simulink model "P4_Model_2"  (R2023b)
settings: Solver=VariableStepAuto  StartTime=0.0  StopTime=10.0  RelTol=1e-3
values from neighbouring files (symbols this model uses):
  C0 = 0.0041    [Finalinit.m]
  C1 = 0.000066    (= 6.6e-05)    [Finalinit.m]
  C2 = 0.5*Rho*A*Cd    (= 0.51156)    [Finalinit.m]
  Iw = 0.5*7*(r^2)    (= 0.4536)    [Finalinit.m]
  M = 1000    [Finalinit.m]
  r = 0.36    [Finalinit.m]
  rps2rpm = 60/(2*pi())    [Finalinit.m]
undefined symbols (not defined in the file or in its folder): batData, carData, motorData
libraries: slpidlib x2
settings Model: Creator=jessi  LastModifiedBy=Beye

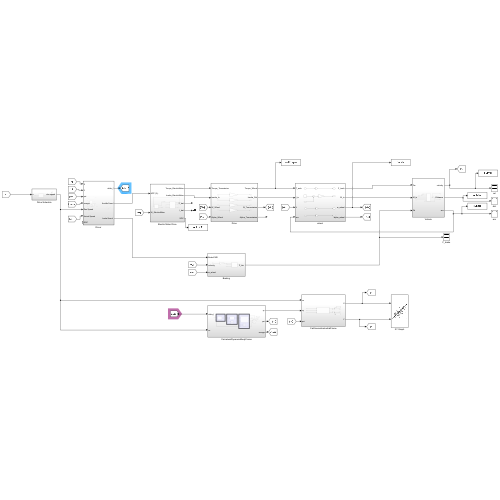
[thumbnail: Simulink's stored preview of the top-level diagram]
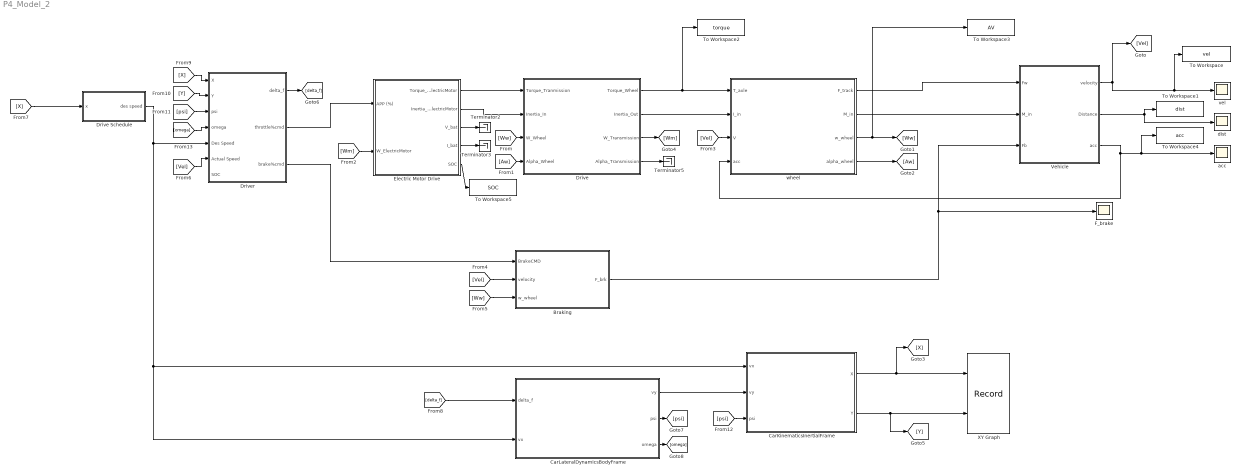
== system P4_Model_2 ==
  Braking : Subsystem
  CarKinematicsInertialFrame : Subsystem
  CarLateralDynamicsBodyFrame : Subsystem
  Drive : Subsystem
  Drive Schedule : Subsystem
  Driver : Subsystem
  Electric Motor Drive : Subsystem
  F_brake : Scope
  Terminator2 : Terminator
  Terminator3 : Terminator
  Terminator5 : Terminator
  To Workspace : ToWorkspace  VariableName=vel  SaveFormat=Timeseries  SampleTime=-1
  To Workspace1 : ToWorkspace  VariableName=dist  SaveFormat=Timeseries  SampleTime=-1
  To Workspace2 : ToWorkspace  VariableName=torque  SaveFormat=Timeseries  SampleTime=-1
  To Workspace3 : ToWorkspace  VariableName=AV  SaveFormat=Timeseries  SampleTime=-1
  To Workspace4 : ToWorkspace  VariableName=acc  SaveFormat=Timeseries  SampleTime=-1
  To Workspace5 : ToWorkspace  VariableName=SOC  SaveFormat=Timeseries  SampleTime=-1
  Vehicle : Subsystem
  XY Graph : Record  FileSettingsInternal="{\"entries\":[{\"content\":{\"excelSettings\":{\"content\":{},\"type\":\"Streamout.ExcelSettings\"}},\"type\":\"Streamout.FileSettingStorage\",\"uuid\":\"\"}],\"packageUris\":[\"http:\\/\\/schema.mathworks.com\\/mf0\\/streamout_blocks\\/R2020a\"],\"version\":\"1.0\"}"  Layout=[1 1]  SignalsInternal="{\"entries\":[{\"content\":{\"signals\":[{\"content\":{\"blockPath\":[],\"dimensions\":[1],\"domain\":\"\",\"lineColor\":\"#0072bd\",\"port\":1,\"sid\":[\"\"],\"signalID\":785,\"signalName\":\"CarKinematicsInertialFrame:1\"},\"type\":\"RecordBlkView.Signal\",\"uuid\":\"\"},{\"content\":{\"blockPath\":[],\"dimensions\":[1],\"domain\":\"\",\"lineColor\":\"#d95319\",\"port\":2,\"sid\":[\"\"],\"signalID\":789,\"signalName\":\"CarKinematicsInertialFrame:2\"},\"type\":\"RecordBlkView.Signal\",\"uuid\":\"\"}]},\"type\":\"RecordBlkView.InputSignals\",\"uuid\":\"\"}],\"packageUris\":[\"http:\\/\\/schema.mathworks.com\\/mf0\\/streamout_blocks\\/R2020a\"],\"version\":\"1.0\"}"  VisualizationBindings="{\"xyplotplugin\":{\"info\":[{\"series\":[],\"subplotID\":1}]}}"  CompatibilityTag=XY  st=-1
  acc : Scope
  dist : Scope
  vel : Scope
  "wheel " : Subsystem
  wires:
  [Ww] -> Braking/3(w_wheel)
  [Vel] -> Braking/2("velocity ")
  "wheel "/3(w_wheel) -> To Workspace3/1, [Ww]
  "wheel "/1(F_track) -> Vehicle/1("Fw ")
  [Wm] -> Electric Motor Drive/2(W_ElectricMotor)
  "wheel "/2(M_in) -> Vehicle/2("M_in ")
  [Ww] -> Drive/3(W_Wheel)
  Drive/1(Torque_Wheel) -> To Workspace2/1, "wheel "/1(T_axle)
  Drive/2(Inertia_Out) -> "wheel "/2(I_in)
  Electric Motor Drive/4(I_bat) -> Terminator3/1
  [Vel] -> "wheel "/3(V)
  Electric Motor Drive/5(SOC) -> To Workspace5/1
  Electric Motor Drive/3(V_bat) -> Terminator2/1
  Vehicle/2("Distance ") -> dist/1, To Workspace1/1
  Braking/1("F_brk ") -> F_brake/1, Vehicle/3("Fb ")
  Drive/4(Alpha_Transmission) -> Terminator5/1
  Electric Motor Drive/2(Inertia_ElectricMotor) -> Drive/2(Inertia_In)
  Vehicle/3(acc) -> "wheel "/4(acc), To Workspace4/1, acc/1
  Vehicle/1("velocity ") -> To Workspace/1, vel/1, [Vel]
  Electric Motor Drive/1(Torque_ElectricMotor) -> Drive/1(Torque_Tranmission)
  "wheel "/4(alpha_wheel) -> [Aw]
  [Aw] -> Drive/4(Alpha_Wheel)
  Drive/3(W_Transmission) -> [Wm]
  Drive Schedule/1("des speed ") -> CarKinematicsInertialFrame/1(vx), CarLateralDynamicsBodyFrame/2(vx), Driver/5("Des Speed ")
  [delta_f] -> CarLateralDynamicsBodyFrame/1(delta_f)
  CarKinematicsInertialFrame/1(X) -> [X], XY Graph/1
  CarKinematicsInertialFrame/2(Y) -> [Y], XY Graph/2
  CarLateralDynamicsBodyFrame/1(vy) -> CarKinematicsInertialFrame/2(vy)
  [X] -> Drive Schedule/1(x)
  CarLateralDynamicsBodyFrame/3(omega) -> [omega]
  [Vel] -> Driver/6(Actual Speed)
  [X] -> Driver/1(X)
  [Y] -> Driver/2(Y)
  Driver/1(delta_f) -> [delta_f]
  Driver/3("brake%cmd ") -> Braking/1("BrakeCMD ")
  Driver/2(throttle%cmd) -> Electric Motor Drive/1(APP (%))
  [psi] -> Driver/3(psi)
  CarLateralDynamicsBodyFrame/2(psi) -> [psi]
  [psi] -> CarKinematicsInertialFrame/3(psi)
  [omega] -> Driver/4(omega)

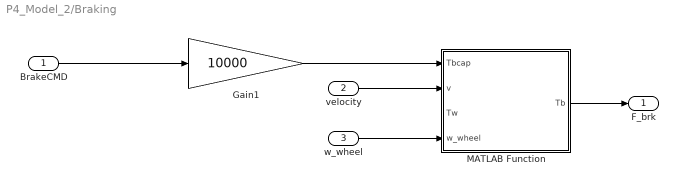
== system P4_Model_2/Braking ==
  "BrakeCMD " : Inport
  "velocity " : Inport  Port=2
  w_wheel : Inport  Port=3
  Gain1 : Gain  Gain=10000
  MATLAB Function : MATLAB Function  TreatAsAtomicUnit=on
  "F_brk " : Outport  VectorParamsAs1DForOutWhenUnconnected=off
  wires:
  "BrakeCMD "/1 -> Gain1/1
  Gain1/1 -> MATLAB Function/1(Tbcap)
  MATLAB Function/1(Tb) -> "F_brk "/1
  "velocity "/1 -> MATLAB Function/2(v)
  w_wheel/1 -> MATLAB Function/4(w_wheel)

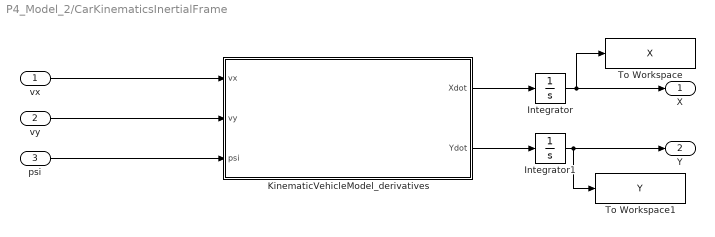
== system P4_Model_2/CarKinematicsInertialFrame ==
  vx : Inport
  vy : Inport  Port=2
  psi : Inport  Port=3
  Integrator : Integrator  InitialCondition=carData.init.X0
  Integrator1 : Integrator  InitialCondition=carData.init.Y0
  KinematicVehicleModel_derivatives : MATLAB Function  TreatAsAtomicUnit=on  mask{obj=carData}
      mask prompts: obj "obj structure"
  To Workspace : ToWorkspace  VariableName=X  SaveFormat=Timeseries  SampleTime=-1
  To Workspace1 : ToWorkspace  VariableName=Y  SaveFormat=Timeseries  SampleTime=-1
  X : Outport
  Y : Outport  Port=2
  wires:
  KinematicVehicleModel_derivatives/1(Xdot) -> Integrator/1
  KinematicVehicleModel_derivatives/2(Ydot) -> Integrator1/1
  Integrator/1 -> To Workspace/1, X/1
  Integrator1/1 -> To Workspace1/1, Y/1
  vx/1 -> KinematicVehicleModel_derivatives/1(vx)
  vy/1 -> KinematicVehicleModel_derivatives/2(vy)
  psi/1 -> KinematicVehicleModel_derivatives/3(psi)

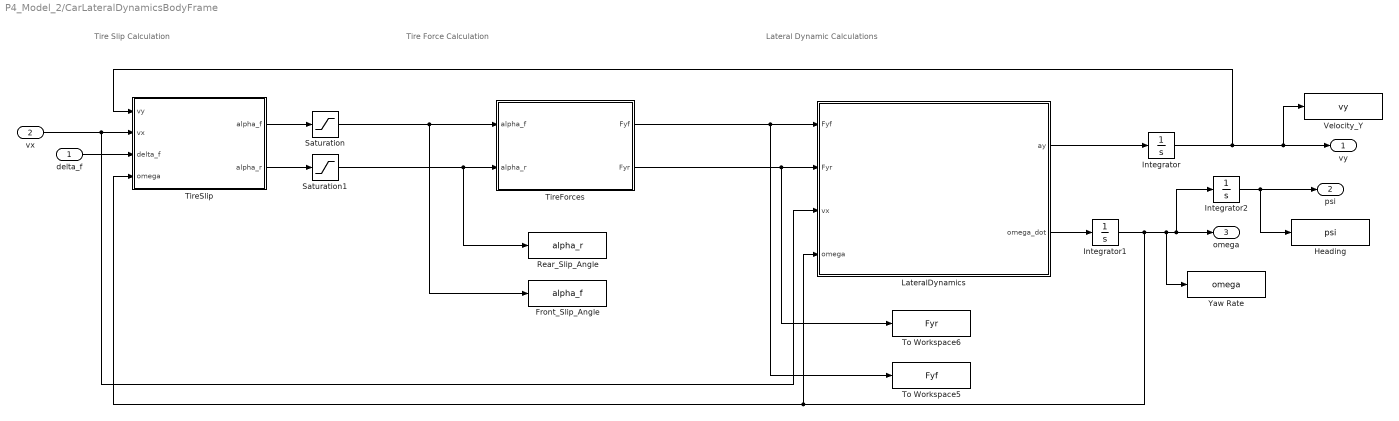
== system P4_Model_2/CarLateralDynamicsBodyFrame ==
  note: Tire Slip Calculation
  note: Tire Force Calculation
  note: Lateral Dynamic Calculations
  delta_f : Inport
  vx : Inport  Port=2
  Front_Slip_Angle : ToWorkspace  VariableName=alpha_f  SaveFormat=Timeseries  SampleTime=-1
  Heading : ToWorkspace  VariableName=psi  SaveFormat=Timeseries  SampleTime=-1
  Integrator : Integrator  InitialCondition=carData.init.vy0
  Integrator1 : Integrator  InitialCondition=carData.init.omega0
  Integrator2 : Integrator  InitialCondition=carData.init.psi0
  LateralDynamics : MATLAB Function  TreatAsAtomicUnit=on  mask{obj=carData}
      mask prompts: obj "obj structure"
  Rear_Slip_Angle : ToWorkspace  VariableName=alpha_r  SaveFormat=Timeseries  SampleTime=-1
  Saturation : Saturate  UpperLimit=carData.maxAlpha  LowerLimit=-carData.maxAlpha
  Saturation1 : Saturate  UpperLimit=carData.maxAlpha  LowerLimit=-carData.maxAlpha
  TireForces : MATLAB Function  TreatAsAtomicUnit=on  mask{obj=carData}
      mask prompts: obj "obj structure"
  TireSlip : MATLAB Function  TreatAsAtomicUnit=on  mask{obj=carData}
      mask prompts: obj "obj structure"
  To Workspace5 : ToWorkspace  VariableName=Fyf  SaveFormat=Timeseries  SampleTime=-1
  To Workspace6 : ToWorkspace  VariableName=Fyr  SaveFormat=Timeseries  SampleTime=-1
  Velocity_Y : ToWorkspace  VariableName=vy  SaveFormat=Timeseries  SampleTime=-1
  Yaw Rate : ToWorkspace  VariableName=omega  SaveFormat=Timeseries  SampleTime=-1
  vy : Outport
  psi : Outport  Port=2
  omega : Outport  Port=3
  wires:
  LateralDynamics/1(ay) -> Integrator/1
  Integrator/1 -> vy/1, Velocity_Y/1, TireSlip/1(vy)
  LateralDynamics/2(omega_dot) -> Integrator1/1
  Integrator1/1 -> Integrator2/1, omega/1, Yaw Rate/1, LateralDynamics/4(omega), TireSlip/4(omega)
  TireSlip/1(alpha_f) -> Saturation/1
  TireSlip/2(alpha_r) -> Saturation1/1
  TireForces/1(Fyf) -> LateralDynamics/1(Fyf), To Workspace5/1
  TireForces/2(Fyr) -> LateralDynamics/2(Fyr), To Workspace6/1
  Saturation/1 -> TireForces/1(alpha_f), Front_Slip_Angle/1
  Saturation1/1 -> TireForces/2(alpha_r), Rear_Slip_Angle/1
  vx/1 -> TireSlip/2(vx), LateralDynamics/3(vx)
  delta_f/1 -> TireSlip/3(delta_f)
  Integrator2/1 -> Heading/1, psi/1

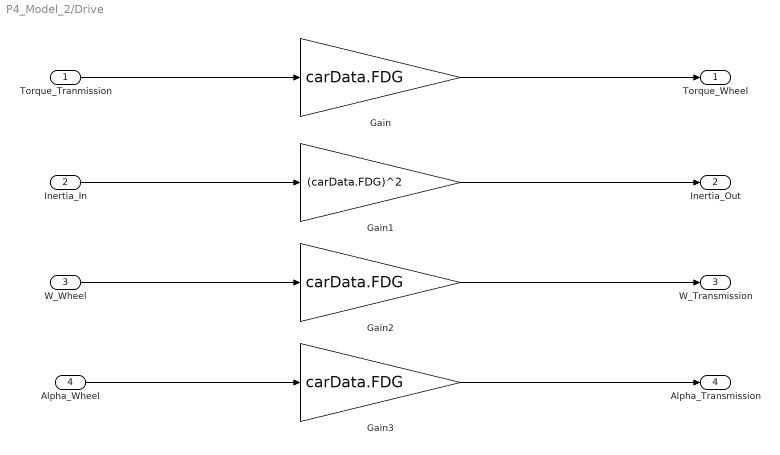
== system P4_Model_2/Drive ==
  Torque_Tranmission : Inport
  Inertia_In : Inport  Port=2
  W_Wheel : Inport  Port=3
  Alpha_Wheel : Inport  Port=4
  Gain : Gain  Gain=carData.FDG
  Gain1 : Gain  Gain=(carData.FDG)^2
  Gain2 : Gain  Gain=carData.FDG
  Gain3 : Gain  Gain=carData.FDG
  Torque_Wheel : Outport
  Inertia_Out : Outport  Port=2
  W_Transmission : Outport  Port=3
  Alpha_Transmission : Outport  Port=4
  wires:
  Torque_Tranmission/1 -> Gain/1
  Inertia_In/1 -> Gain1/1
  W_Wheel/1 -> Gain2/1
  Alpha_Wheel/1 -> Gain3/1
  Gain/1 -> Torque_Wheel/1
  Gain1/1 -> Inertia_Out/1
  Gain2/1 -> W_Transmission/1
  Gain3/1 -> Alpha_Transmission/1

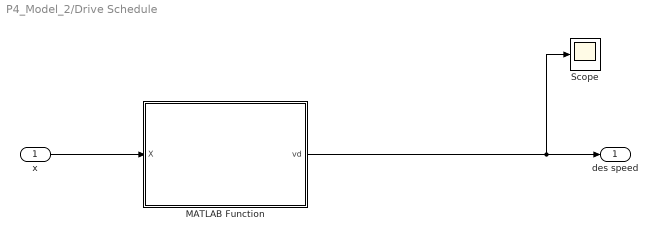
== system P4_Model_2/Drive Schedule ==
  x : Inport
  MATLAB Function : MATLAB Function  TreatAsAtomicUnit=on
  Scope : Scope
  "des speed " : Outport  VectorParamsAs1DForOutWhenUnconnected=off
  wires:
  x/1 -> MATLAB Function/1(X)
  MATLAB Function/1(vd) -> "des speed "/1, Scope/1

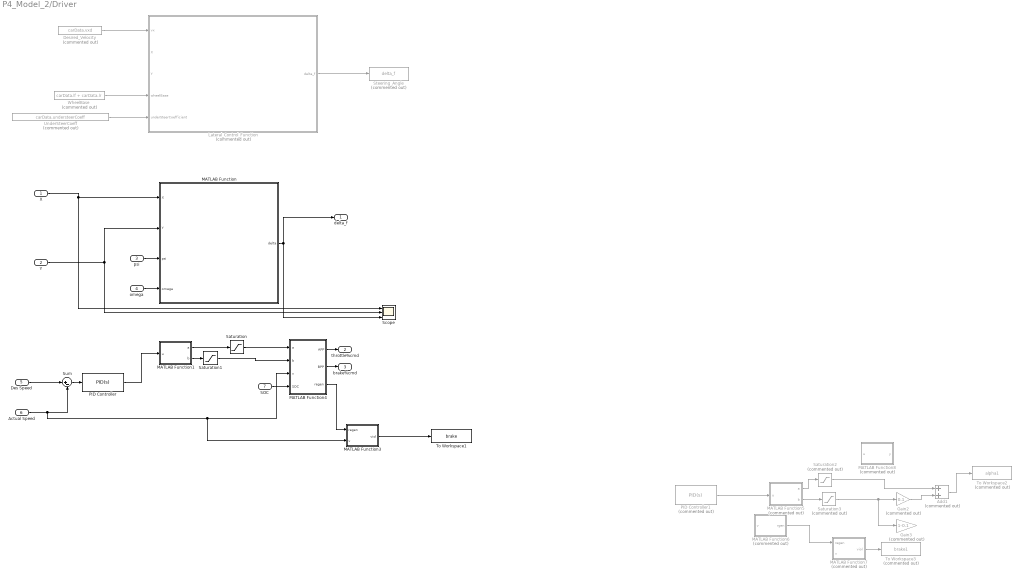
== system P4_Model_2/Driver ==
  X : Inport
  Y : Inport  Port=2
  psi : Inport  Port=3
  omega : Inport  Port=4
  "Des Speed " : Inport  Port=5
  Actual Speed : Inport  Port=6
  SOC : Inport  Port=7
  Add1 : Sum  Commented=on
  Desired_Velocity : Constant  Commented=on  Value=carData.vxd
  Gain2 : Gain  Commented=on  Gain=0.1
  Gain3 : Gain  Commented=on  Gain=1-0.1
  Lateral_Control_Function : MATLAB Function  Commented=on  TreatAsAtomicUnit=on
  MATLAB Function : MATLAB Function  TreatAsAtomicUnit=on
  MATLAB Function1 : MATLAB Function  TreatAsAtomicUnit=on
  MATLAB Function3 : MATLAB Function  TreatAsAtomicUnit=on
  MATLAB Function4 : MATLAB Function  TreatAsAtomicUnit=on
  MATLAB Function5 : MATLAB Function  Commented=on  TreatAsAtomicUnit=on
  MATLAB Function6 : MATLAB Function  Commented=on  TreatAsAtomicUnit=on
  MATLAB Function7 : MATLAB Function  Commented=on  TreatAsAtomicUnit=on
  MATLAB Function8 : MATLAB Function  Commented=on  TreatAsAtomicUnit=on
  PID Controller : slpidlib/PID Controller  Controller=PID  Form=Parallel  TimeDomain=Continuous-time  UseExternalTs=off  SampleTime=-1  IntegratorMethod=Forward Euler  FilterMethod=Forward Euler  ControllerParametersSource=internal  P=0.55  I=0  UseKiTs=off  D=0  N=100  UseFilter=on  TunerSelectOption=Transfer Function Based (PID Tuner App)  InitialConditionSource=internal  InitialConditionForIntegrator=0  InitialConditionForFilter=0  DifferentiatorICPrevScaledInput=0  ExternalReset=none  TrackingMode=off  Kt=1  LimitOutput=on  SatLimitsSource=internal  UpperSaturationLimit=1  LowerSaturationLimit=-1  LinearizeAsGain=off  AntiWindupMode=none  Kb=1  LimitIntegrator=off  UpperIntegratorSaturationLimit=inf  LowerIntegratorSaturationLimit=-inf  POutMin=[]  POutMax=[]  IOutMin=[]  IOutMax=[]  DOutMin=[]  DOutMax=[]  NOutMin=[]  NOutMax=[]  SumOutMin=[]  SumOutMax=[]  SaturationOutMin=[]  SaturationOutMax=[]  PParamMin=[]  PParamMax=[]  IParamMin=[]  IParamMax=[]  DParamMin=[]  DParamMax=[]  NParamMin=[]  NParamMax=[]  KbParamMin=[]  KbParamMax=[]  KtParamMin=[]  KtParamMax=[]  KbOutMin=[]  KbOutMax=[]  KtOutMin=[]  KtOutMax=[]  IntegratorOutMin=[]  IntegratorOutMax=[]  FilterOutMin=[]  FilterOutMax=[]  SumI1OutMin=[]  SumI1OutMax=[]  SumI2OutMin=[]  SumI2OutMax=[]  SumI3OutMin=[]  SumI3OutMax=[]  SumI4OutMin=[]  SumI4OutMax=[]  SumDOutMin=[]  SumDOutMax=[]  DifferentiatorOutMin=[]  DifferentiatorOutMax=[]  FilterDiffOutCoefMin=[]  FilterDiffOutCoefMax=[]  ReciprocalOutMin=[]  ReciprocalOutMax=[]  SumDenOutMin=[]  SumDenOutMax=[]  SumNumOutMin=[]  SumNumOutMax=[]  DivideOutMin=[]  DivideOutMax=[]  UdiffTsProdOutMin=[]  UdiffTsProdOutMax=[]  NTsProdOutMin=[]  NTsProdOutMax=[]  UintegralTsProdOutMin=[]  UintegralTsProdOutMax=[]  UngainTsProdOutMin=[]  UngainTsProdOutMax=[]  ClampingZeroOutDataTypeStr=Inherit: Inherit via back propagation  ClampingZeroOutMin=[]  ClampingZeroOutMax=[]  FilterDenConstantOutDataTypeStr=Inherit: Inherit via back propagation  FilterDenConstantOutMin=[]  FilterDenConstantOutMax=[]  PCopyOutDataTypeStr=Inherit: Inherit via back propagation  PCopyOutMin=[]  PCopyOutMax=[]  NCopyOutDataTypeStr=Inherit: Inherit via back propagation  NCopyOutMin=[]  NCopyOutMax=[]  IntegratorContinuousStateAttributes=''  IntegratorStateMustResolveToSignalObject=off  IntegratorRTWStateStorageClass=Auto  FilterContinuousStateAttributes=''  FilterStateMustResolveToSignalObject=off  FilterRTWStateStorageClass=Auto  ParallelPVariant=InternalParameters  IdealPVariant=Disabled  IVariant=InternalParameters  DVariant=InternalParameters  IntegratorVariant=Continuous  SatVariant=Enabled  AWVariant=Passthrough  PCopyVariant=Disabled  TRVariant=Disabled  FdbkBlocksVariant=Forward  IdealPFdbkVariant=Disabled  SatFdbkVariant=Disabled  DerivativeFilterVariant=ContFilter  NVariant=InternalParameters  NCopyVariant=Disabled  FilterICVariant=InternalICsFilter  IntegratorICVariant=InternalICs  ExternalResetVariant=Disabled  TRSumVariant=Passthrough  SumFdbkVariant=Disabled  SumVariant=Sum_PID  TsampFilterVariant=InternalTs  TsampNgainVariant=Passthrough  TsampIntegralVariant=Disabled_SignalSpec  ExternalSaturationOutDataTypeStr=Inherit: Same as second input
  PID Controller1 : slpidlib/PID Controller  Commented=on  Controller=PID  Form=Parallel  TimeDomain=Continuous-time  UseExternalTs=off  SampleTime=-1  IntegratorMethod=Forward Euler  FilterMethod=Forward Euler  ControllerParametersSource=internal  P=0.55  I=0  UseKiTs=off  D=0  N=100  UseFilter=on  TunerSelectOption=Transfer Function Based (PID Tuner App)  InitialConditionSource=internal  InitialConditionForIntegrator=0  InitialConditionForFilter=0  DifferentiatorICPrevScaledInput=0  ExternalReset=none  TrackingMode=off  Kt=1  LimitOutput=on  SatLimitsSource=internal  UpperSaturationLimit=1  LowerSaturationLimit=-1  LinearizeAsGain=off  AntiWindupMode=none  Kb=1  LimitIntegrator=off  UpperIntegratorSaturationLimit=inf  LowerIntegratorSaturationLimit=-inf  POutMin=[]  POutMax=[]  IOutMin=[]  IOutMax=[]  DOutMin=[]  DOutMax=[]  NOutMin=[]  NOutMax=[]  SumOutMin=[]  SumOutMax=[]  SaturationOutMin=[]  SaturationOutMax=[]  PParamMin=[]  PParamMax=[]  IParamMin=[]  IParamMax=[]  DParamMin=[]  DParamMax=[]  NParamMin=[]  NParamMax=[]  KbParamMin=[]  KbParamMax=[]  KtParamMin=[]  KtParamMax=[]  KbOutMin=[]  KbOutMax=[]  KtOutMin=[]  KtOutMax=[]  IntegratorOutMin=[]  IntegratorOutMax=[]  FilterOutMin=[]  FilterOutMax=[]  SumI1OutMin=[]  SumI1OutMax=[]  SumI2OutMin=[]  SumI2OutMax=[]  SumI3OutMin=[]  SumI3OutMax=[]  SumI4OutMin=[]  SumI4OutMax=[]  SumDOutMin=[]  SumDOutMax=[]  DifferentiatorOutMin=[]  DifferentiatorOutMax=[]  FilterDiffOutCoefMin=[]  FilterDiffOutCoefMax=[]  ReciprocalOutMin=[]  ReciprocalOutMax=[]  SumDenOutMin=[]  SumDenOutMax=[]  SumNumOutMin=[]  SumNumOutMax=[]  DivideOutMin=[]  DivideOutMax=[]  UdiffTsProdOutMin=[]  UdiffTsProdOutMax=[]  NTsProdOutMin=[]  NTsProdOutMax=[]  UintegralTsProdOutMin=[]  UintegralTsProdOutMax=[]  UngainTsProdOutMin=[]  UngainTsProdOutMax=[]  ClampingZeroOutDataTypeStr=Inherit: Inherit via back propagation  ClampingZeroOutMin=[]  ClampingZeroOutMax=[]  FilterDenConstantOutDataTypeStr=Inherit: Inherit via back propagation  FilterDenConstantOutMin=[]  FilterDenConstantOutMax=[]  PCopyOutDataTypeStr=Inherit: Inherit via back propagation  PCopyOutMin=[]  PCopyOutMax=[]  NCopyOutDataTypeStr=Inherit: Inherit via back propagation  NCopyOutMin=[]  NCopyOutMax=[]  IntegratorContinuousStateAttributes=''  IntegratorStateMustResolveToSignalObject=off  IntegratorRTWStateStorageClass=Auto  FilterContinuousStateAttributes=''  FilterStateMustResolveToSignalObject=off  FilterRTWStateStorageClass=Auto  ParallelPVariant=InternalParameters  IdealPVariant=Disabled  IVariant=InternalParameters  DVariant=InternalParameters  IntegratorVariant=Continuous  SatVariant=Enabled  AWVariant=Passthrough  PCopyVariant=Disabled  TRVariant=Disabled  FdbkBlocksVariant=Forward  IdealPFdbkVariant=Disabled  SatFdbkVariant=Disabled  DerivativeFilterVariant=ContFilter  NVariant=InternalParameters  NCopyVariant=Disabled  FilterICVariant=InternalICsFilter  IntegratorICVariant=InternalICs  ExternalResetVariant=Disabled  TRSumVariant=Passthrough  SumFdbkVariant=Disabled  SumVariant=Sum_PID  TsampFilterVariant=InternalTs  TsampNgainVariant=Passthrough  TsampIntegralVariant=Disabled_SignalSpec  ExternalSaturationOutDataTypeStr=Inherit: Same as second input
  Saturation : Saturate  UpperLimit=1  LowerLimit=0
  Saturation1 : Saturate  UpperLimit=0  LowerLimit=-1
  Saturation2 : Saturate  Commented=on  UpperLimit=1  LowerLimit=0
  Saturation3 : Saturate  Commented=on  UpperLimit=0  LowerLimit=-1
  Scope : Scope  NumInputPorts=3
  Steering_Angle : ToWorkspace  Commented=on  VariableName=delta_f  SaveFormat=Timeseries  SampleTime=-1
  Sum : Sum  Inputs=|+-
  To Workspace1 : ToWorkspace  VariableName=brake  SaveFormat=Timeseries  SampleTime=-1
  To Workspace2 : ToWorkspace  Commented=on  VariableName=alpha1  SaveFormat=Timeseries  SampleTime=-1
  To Workspace3 : ToWorkspace  Commented=on  VariableName=brake1  SaveFormat=Timeseries  SampleTime=-1
  UnderSteerCoeff : Constant  Commented=on  Value=carData.understeerCoeff
  WheelBase : Constant  Commented=on  Value=carData.lf + carData.lr
  delta_f : Outport
  throttle%cmd : Outport  Port=2
  "brake%cmd " : Outport  Port=3
  wires:
  Desired_Velocity/1 -> Lateral_Control_Function/1(vx)
  WheelBase/1 -> Lateral_Control_Function/4(wheelBase)
  Lateral_Control_Function/1(delta_f) -> Steering_Angle/1
  UnderSteerCoeff/1 -> Lateral_Control_Function/5(underSteerCoefficient)
  MATLAB Function/1(delta) -> delta_f/1, Scope/3
  X/1 -> Scope/1, MATLAB Function/1(X)
  Y/1 -> Scope/2, MATLAB Function/2(Y)
  psi/1 -> MATLAB Function/3(psi)
  omega/1 -> MATLAB Function/4(omega)
  PID Controller/1 -> MATLAB Function1/1(u)
  MATLAB Function1/2(b) -> Saturation1/1
  Actual Speed/1 -> MATLAB Function3/2(v), MATLAB Function4/3(v), Sum/2
  Sum/1 -> PID Controller/1
  MATLAB Function1/1(a) -> Saturation/1
  "Des Speed "/1 -> Sum/1
  MATLAB Function3/1(viol) -> To Workspace1/1
  MATLAB Function6/1(rgen) -> MATLAB Function7/1(regen)
  Gain2/1 -> Add1/2
  Saturation3/1 -> Gain3/1, Gain2/1
  ? -> PID Controller1/1
  PID Controller1/1 -> MATLAB Function5/1(u)
  Add1/1 -> To Workspace2/1
  Saturation2/1 -> Add1/1
  MATLAB Function5/2(b) -> Saturation3/1
  MATLAB Function5/1(a) -> Saturation2/1
  MATLAB Function7/1(viol) -> To Workspace3/1
  MATLAB Function4/2(BPP) -> "brake%cmd "/1
  MATLAB Function4/1(APP) -> throttle%cmd/1
  MATLAB Function4/3(regen) -> MATLAB Function3/1(regen)
  Saturation/1 -> MATLAB Function4/1(a)
  Saturation1/1 -> MATLAB Function4/2(b)
  SOC/1 -> MATLAB Function4/4(SOC)

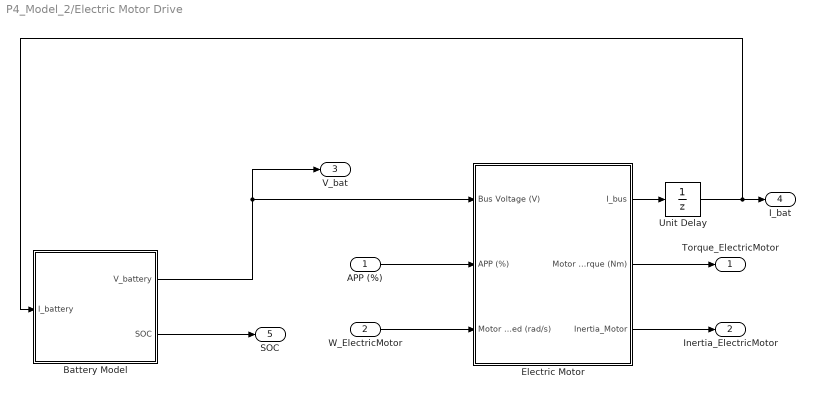
== system P4_Model_2/Electric Motor Drive ==
  APP (%) : Inport
  W_ElectricMotor : Inport  Port=2
  Battery Model : Subsystem  TreatAsAtomicUnit=on
  Electric Motor : Subsystem  TreatAsAtomicUnit=on
  Unit Delay : UnitDelay  SampleTime=-1  HasFrameUpgradeWarning=on
  Torque_ElectricMotor : Outport
  Inertia_ElectricMotor : Outport  Port=2
  V_bat : Outport  Port=3
  I_bat : Outport  Port=4
  SOC : Outport  Port=5
  wires:
  Electric Motor/2(Motor Torque (Nm)) -> Torque_ElectricMotor/1
  Battery Model/2(SOC) -> SOC/1
  Electric Motor/3(Inertia_Motor) -> Inertia_ElectricMotor/1
  W_ElectricMotor/1 -> Electric Motor/3(Motor Speed (rad/s))
  Electric Motor/1(I_bus) -> Unit Delay/1
  APP (%)/1 -> Electric Motor/2(APP (%))
  Battery Model/1(V_battery) -> Electric Motor/1(Bus Voltage (V)), V_bat/1
  Unit Delay/1 -> Battery Model/1(I_battery), I_bat/1

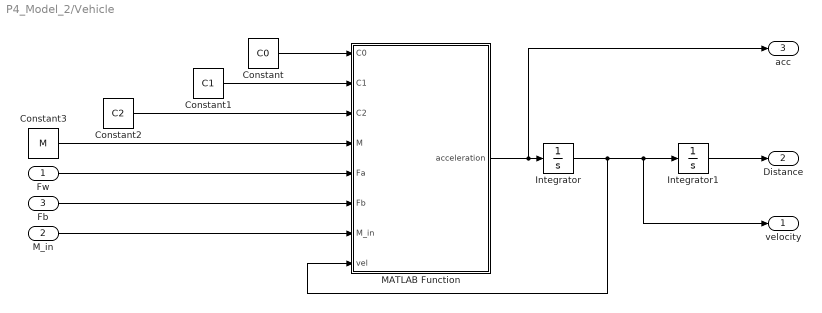
== system P4_Model_2/Vehicle ==
  "Fw " : Inport
  "M_in " : Inport  Port=2
  "Fb " : Inport  Port=3
  Constant : Constant  Value=C0
  Constant1 : Constant  Value=C1
  Constant2 : Constant  Value=C2
  Constant3 : Constant  Value=M
  Integrator : Integrator  LimitOutput=on  LowerSaturationLimit=0
  Integrator1 : Integrator
  MATLAB Function : MATLAB Function  TreatAsAtomicUnit=on
  "velocity " : Outport  VectorParamsAs1DForOutWhenUnconnected=off
  "Distance " : Outport  Port=2  VectorParamsAs1DForOutWhenUnconnected=off
  acc : Outport  Port=3
  wires:
  Constant1/1 -> MATLAB Function/2(C1)
  Constant/1 -> MATLAB Function/1(C0)
  MATLAB Function/1(acceleration) -> acc/1, Integrator/1
  Constant2/1 -> MATLAB Function/3(C2)
  Constant3/1 -> MATLAB Function/4(M)
  "Fw "/1 -> MATLAB Function/5(Fa)
  "Fb "/1 -> MATLAB Function/6(Fb)
  Integrator/1 -> MATLAB Function/8(vel), "velocity "/1, Integrator1/1
  Integrator1/1 -> "Distance "/1
  "M_in "/1 -> MATLAB Function/7(M_in)

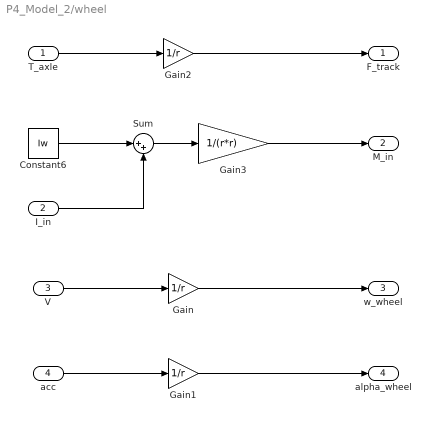
== system P4_Model_2/wheel  ==
  T_axle : Inport
  I_in : Inport  Port=2
  V : Inport  Port=3
  acc : Inport  Port=4
  Constant6 : Constant  Value=Iw
  Gain : Gain  Gain=1/r
  Gain1 : Gain  Gain=1/r
  Gain2 : Gain  Gain=1/r
  Gain3 : Gain  Gain=1/(r*r)
  Sum : Sum  Inputs=|++
  F_track : Outport
  M_in : Outport  Port=2
  w_wheel : Outport  Port=3
  alpha_wheel : Outport  Port=4
  wires:
  Gain/1 -> w_wheel/1
  V/1 -> Gain/1
  acc/1 -> Gain1/1
  Gain1/1 -> alpha_wheel/1
  T_axle/1 -> Gain2/1
  Gain2/1 -> F_track/1
  Gain3/1 -> M_in/1
  Constant6/1 -> Sum/1
  I_in/1 -> Sum/2
  Sum/1 -> Gain3/1

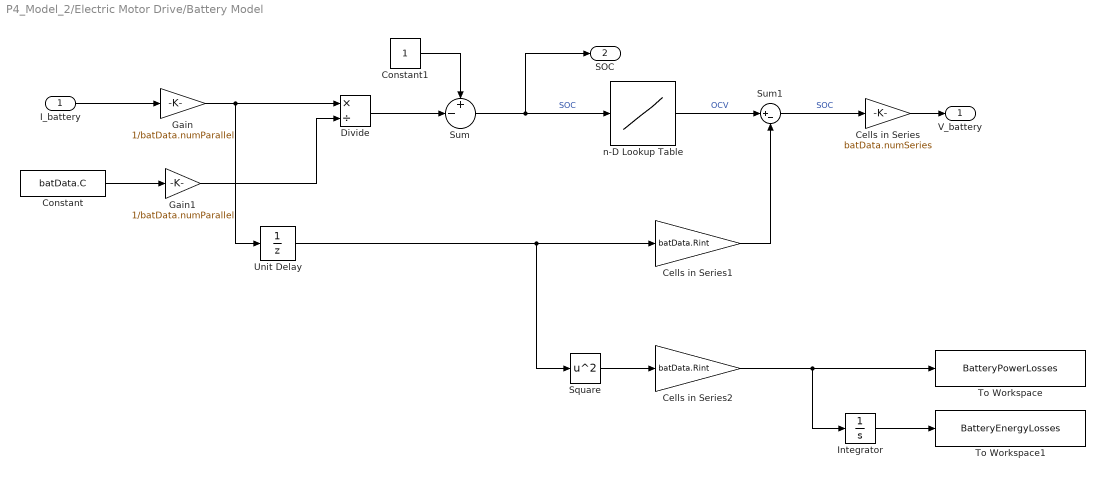
== system P4_Model_2/Electric Motor Drive/Battery Model ==
  I_battery : Inport
  Cells in Series : Gain  Gain=batData.numSeries
  Cells in Series1 : Gain  Gain=batData.Rint
  Cells in Series2 : Gain  Gain=batData.Rint
  Constant : Constant  Value=batData.C
  Constant1 : Constant
  Divide : Product  Inputs=*/
  Gain : Gain  Gain=1/batData.numParallel
  Gain1 : Gain  Gain=1/batData.numParallel
  Integrator : Integrator
  Square : Math  Operator=square
  Sum : Sum  Inputs=+-|
  Sum1 : Sum  Inputs=|+-
  To Workspace : ToWorkspace  VariableName=BatteryPowerLosses  SaveFormat=Timeseries  SampleTime=-1
  To Workspace1 : ToWorkspace  VariableName=BatteryEnergyLosses  SaveFormat=Timeseries  SampleTime=-1
  Unit Delay : UnitDelay  SampleTime=-1  HasFrameUpgradeWarning=on
  n-D Lookup Table : Lookup_n-D  NumberOfTableDimensions=1  BreakpointsForDimension1=batData.SOC  BreakpointsForDimension3=[5, 7]  Table=batData.OCV  InternalRulePriority=Speed  RndMeth=Simplest
  V_battery : Outport
  SOC : Outport  Port=2
  wires:
  I_battery/1 -> Gain/1
  Gain/1 -> Unit Delay/1, Divide/1
  Gain1/1 -> Divide/2
  Constant/1 -> Gain1/1
  Constant1/1 -> Sum/1
  Divide/1 -> Sum/2
  Sum/1 -> SOC/1, n-D Lookup Table/1  "SOC"
  n-D Lookup Table/1 -> Sum1/1  "OCV"
  Cells in Series/1 -> V_battery/1
  Sum1/1 -> Cells in Series/1  "SOC"
  Cells in Series1/1 -> Sum1/2
  Square/1 -> Cells in Series2/1
  Cells in Series2/1 -> Integrator/1, To Workspace/1
  Integrator/1 -> To Workspace1/1
  Unit Delay/1 -> Square/1, Cells in Series1/1

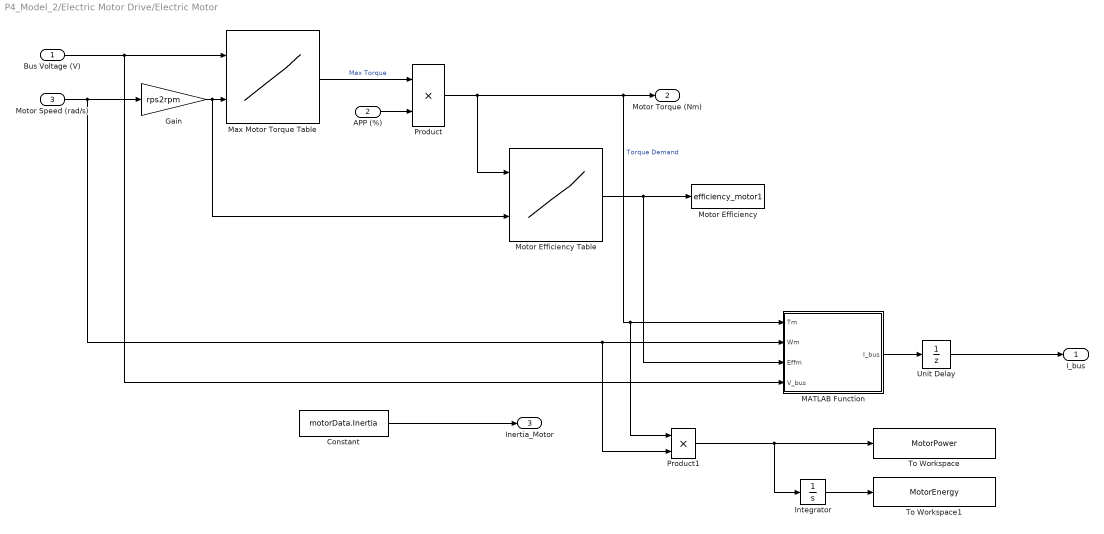
== system P4_Model_2/Electric Motor Drive/Electric Motor ==
  Bus Voltage (V) : Inport
  APP (%) : Inport  Port=2
  Motor Speed (rad/s) : Inport  Port=3
  Constant : Constant  Value=motorData.Inertia
  Gain : Gain  Gain=rps2rpm
  Integrator : Integrator
  MATLAB Function : MATLAB Function  TreatAsAtomicUnit=on
  Max Motor Torque Table : Lookup_n-D  BreakpointsForDimension1=motorData.vbus  BreakpointsForDimension2=motorData.rpm  BreakpointsForDimension3=[5, 7]  Table=motorData.maxtorque  InternalRulePriority=Speed  RndMeth=Simplest
      settings: InputPortMap=u0,u1
  Motor Efficiency : ToWorkspace  VariableName=efficiency_motor1  SaveFormat=Timeseries  SampleTime=-1
  Motor Efficiency Table : Lookup_n-D  BreakpointsForDimension1=motorData.eta_torque  BreakpointsForDimension2=motorData.eta_speed  BreakpointsForDimension3=[5, 7]  Table=motorData.eta_val  InternalRulePriority=Speed  RndMeth=Simplest
      settings: InputPortMap=u0,u1
  Product : Product
  Product1 : Product
  To Workspace : ToWorkspace  VariableName=MotorPower  SaveFormat=Timeseries  SampleTime=-1
  To Workspace1 : ToWorkspace  VariableName=MotorEnergy  SaveFormat=Timeseries  SampleTime=-1
  Unit Delay : UnitDelay  SampleTime=-1  HasFrameUpgradeWarning=on
  I_bus : Outport
  Motor Torque (Nm) : Outport  Port=2
  Inertia_Motor : Outport  Port=3
  wires:
  Constant/1 -> Inertia_Motor/1
  APP (%)/1 -> Product/2
  Max Motor Torque Table/1 -> Product/1  "Max Torque"
  Product/1 -> Motor Efficiency Table/1, Product1/1, MATLAB Function/1(Tm), Motor Torque (Nm)/1  "Torque Demand"
  Gain/1 -> Motor Efficiency Table/2, Max Motor Torque Table/2
  Motor Speed (rad/s)/1 -> Gain/1, Product1/2, MATLAB Function/2(Wm)
  Motor Efficiency Table/1 -> MATLAB Function/3(Effm), Motor Efficiency/1
  Integrator/1 -> To Workspace1/1
  Product1/1 -> Integrator/1, To Workspace/1
  MATLAB Function/1(I_bus) -> Unit Delay/1
  Unit Delay/1 -> I_bus/1
  Bus Voltage (V)/1 -> MATLAB Function/4(V_bus), Max Motor Torque Table/1

== matlab function P4_Model_2/Driver/Lateral_Control_Function ==
  data: vx input; delta_f output; X input; Y input; wheelBase input; underSteerCoefficient input
function delta_f   = latControl(vx,X,Y,wheelBase, underSteerCoefficient)

track_radius = 200;
track_length = 900;

track_seg1_x0 = 0;
track_seg1_y0 = 0;
track_seg1_x1 = track_length;
track_seg1_y1 = 0;
track_seg2_x0 = track_seg1_x1;
track_seg2_y0 = track_seg1_y1;
track_seg2_x1 = track_seg2_x0;
track_seg2_y1 = track_seg2_y0 + 2 * track_radius;
track_seg3_x0 = track_seg2_x1;
track_seg3_y0 = track_seg2_y1;
track_seg3_x1 = track_seg3_x0 - track_length;
track_seg3_y1 = track_seg3_y0;
track_seg4_x0 = track_seg3_x1;
track_seg4_y0 = track_seg3_y1;
track_seg4_x1 = track_seg1_x0;
track_seg4_y1 = track_seg1_y0;

if X > track_seg1_x0
    if X > track_seg1_x1
        segment = 2;
    else
        if Y > (track_seg2_y0 + track_seg2_y1)/2
            segment = 3;
        else
            segment = 1;
        end
    end
else
    segment = 4;
end



switch(segment)
    case 1
        delta_f = 0;
    case 2
        delta_f = - (wheelBase / track_radius + 1 * underSteerCoefficient * vx^2);
    case 3
        delta_f = 0;
    case 4
        delta_f = - (wheelBase / track_radius + 1 * underSteerCoefficient * vx^2);
    otherwise
        delta_f = 0;
end

== matlab function P4_Model_2/Driver/MATLAB Function ==
  data: X input; delta output; Y input; psi input; omega input
function delta = SimplestDriver(X,Y,psi,omega)

if X > 900
    R = 200;
    L = pi*R;
    delta = L/R;
    
     
elseif X < 0
    R = 200;
    L = pi*R;
    delta = L/R;
    
elseif X < 900 && Y < 1
    delta = 0;


elseif X < 900 && X > 850 && Y > 390
    k = -0.00040;
    psi_d = 0;

    delta = k*(psi-psi_d);

else
    k = -0.00012;
    psi_d = 3;

    delta = k*(psi-psi_d);
end

== matlab function P4_Model_2/Driver/MATLAB Function1 ==
  data: u input; a output; b output
% Checks if there is a difference between actual speed and desired speed

% u is calculated using the sum function in the simulink model

function [a,b] = fcn(u)

if u>0 % If the difference is greater than zero, then we need to speed up since actual speed is less than desired speed
    acc=u; % We send how much we need to speed up to the throttle command
    brk=0; % Do nothing for the break command
elseif u<0 % If the difference is less than zero, then we need to slow down since the actual speed is less than the desired speed
    acc=0; % Do nothing for throttle command
    brk=-u; % We send how much we need to break to the break command
else % If the desired and actual speed is the same
    acc=0; % Do nothing for throttle command
    brk=0; % Do nothing for the break command
end
a= acc; % storing how much acceleration required to a
b= brk; % storing how much break acceleration required to b

== matlab function P4_Model_2/Driver/MATLAB Function3 ==
  data: regen input; viol output; v input
function viol = violfcn(regen, v)
    speed = v;
    if speed < 5
        regen_vio = 0;
        if abs(regen - regen_vio) < 1e-6
            viol = 0;
        else
            viol = 1;
        end

    elseif speed == 25
        regen_vio = 0.95;
        if abs(regen - regen_vio) < 1e-6
            viol = 0;
        else
            viol = 1;
        end

    elseif v > 25
        regen_vio = 0.95;
        if abs(regen - regen_vio) < 1e-6
            viol = 0;
        else
            viol = 1;
        end
    else
        regen_vio = ((0.95/20)*speed) - 0.2375;
        % disp(regen_vio);
        % disp(regen);
        if abs(regen - regen_vio) < 1e-6
            viol = 0;
        else
            viol = 1;
        end
    end

== matlab function P4_Model_2/Driver/MATLAB Function4 ==
  data: a input; APP output; BPP output; b input; v input; SOC input; regen output
function [APP, BPP, regen] = fcn(a, b, v, SOC)
    % Convert velocity to mph from m/s
    speed = v * (3600 / 1600);

    % Calculate regen based on speed and braking command
    regen = calculateRegen(speed);

    APP = a + b * regen;  % Add regen to the acceleration command
    BPP = b * (1 - regen);  % Rest is friction braking
end

function regen = calculateRegen(speed)
  if speed < 5
      regen = 0;
  elseif speed == 25
        regen = 0.95;
  elseif speed > 25
      regen = 0.95;
  else
      regen = ((0.95/20)*speed) - 0.2375;
  end 
end

== matlab function P4_Model_2/Driver/MATLAB Function5 ==
  data: u input; a output; b output
% Checks if there is a difference between actual speed and desired speed

% u is calculated using the sum function in the simulink model

function [a,b] = fcn(u)

if u>0 % If the difference is greater than zero, then we need to speed up since actual speed is less than desired speed
    acc=u; % We send how much we need to speed up to the throttle command
    brk=0; % Do nothing for the break command
elseif u<0 % If the difference is less than zero, then we need to slow down since the actual speed is less than the desired speed
    acc=0; % Do nothing for throttle command
    brk=-u; % We send how much we need to break to the break command
else % If the desired and actual speed is the same
    acc=0; % Do nothing for throttle command
    brk=0; % Do nothing for the break command
end
a= acc; % storing how much acceleration required to a
b= brk; % storing how much break acceleration required to b

== matlab function P4_Model_2/Drive Schedule/MATLAB Function ==
  data: X input; vd output
function vd = fcn(X)

if X > 0 && X < 900
    vd = 60;
else
    vd = 10;
end

== matlab function P4_Model_2/Driver/MATLAB Function6 ==
  data: v input; rgen output
function rgen = fcn(v)
if v <= 5
    rgen = 0;

elseif v > 5
    rgen = .0475 * (v-5);

else
    rgen = .95;

end

== matlab function P4_Model_2/Driver/MATLAB Function7 ==
  data: regen input; viol output; v input
function viol = violfcn(regen, v)
    speed = (3600/1600)*v;
    if speed < 5
        regen_vio = 0;
        if regen == regen_vio
            viol = 0;
        else
            viol = 1;
        end

    elseif speed == 25
        regen_vio = 0.95;
        if regen == regen_vio
            viol = 0;
        else
            viol = 1;
        end

    elseif v > 25
        regen_vio = 0.95;
        if regen == regen_vio
            viol = 0;
        else
            viol = 1;
        end
    else
        regen_vio = ((0.95/20)*speed) - 0.2375;
        if regen == regen_vio
            viol = 0;
        else
            viol = 1;
        end
    end

== matlab function P4_Model_2/Driver/MATLAB Function8 ==
  data: u input; y output
function y = fcn(u)

== matlab function P4_Model_2/Vehicle/MATLAB Function ==
  data: C0 input; acceleration output; C1 input; C2 input; M input; Fa input; Fb input; M_in input; vel input
function acceleration   = vehicle(C0,C1,C2,M,Fa,Fb,M_in, vel)

acceleration = (((Fa-Fb))-(C0+ C1*vel + C2*(vel)^2))/(M+M_in);


% Fa: Force from wheel.
% Fb: Force from brake.
% -(C0+ C1*vel + C2*(vel)^2)): Force from drag (opposite direction of motion)

== matlab function P4_Model_2/CarKinematicsInertialFrame/KinematicVehicleModel_derivatives ==
  data: vx input; vy input; psi input size=1; Xdot output; Ydot output
    function [Xdot, Ydot] = fcn(vx, vy, psi)
    temp = TF(psi) * [vx;vy]; 
    Xdot = temp(1);
    Ydot = temp(2);
  
end

function y = TF(psi)
    y = [cos(psi), -sin(psi); sin(psi), cos(psi)];
end

== matlab function P4_Model_2/Electric Motor Drive/Electric Motor/MATLAB Function ==
  data: Tm input; I_bus output; Wm input; Effm input; V_bus input
function I_bus = fcn(Tm,Wm,Effm,V_bus)

%I_bus = (Tm*Wm/Effm)/V_bus;

Pm=Tm*Wm;
    if Pm >= 0
        sgn_m = 1;
    else
        sgn_m = -1;
    end
I_bus = ( (Pm) * (Effm)^(sgn_m) ) / V_bus;

== matlab function P4_Model_2/CarLateralDynamicsBodyFrame/LateralDynamics ==
  data: Fyf input; Fyr input size=1; vx input; omega input; ay output; obj parameter; omega_dot output
function [ay, omega_dot] = fcn(Fyf, Fyr, vx, omega, obj)

Fy = Fyf + Fyr;
ay = Fy / obj.Mass - omega * vx;
        
M  = Fyf * obj.lf - Fyr * obj.lr;        
omega_dot = M / obj.Inertia;        

end

== matlab function P4_Model_2/CarLateralDynamicsBodyFrame/TireForces ==
  data: alpha_f input; alpha_r input; Fyf output; obj parameter; Fyr output
function [Fyf, Fyr] = fcn(alpha_f, alpha_r, obj)

Fyf = min(obj.Fyfmax,obj.Calpha_f * alpha_f);
Fyr = min(obj.Fyrmax, obj.Calpha_r * alpha_r);
end

== matlab function P4_Model_2/Braking/MATLAB Function ==
  data: Tbcap input; Tb output; v input; Tw input; w_wheel input
function Tb = fcn(Tbcap, v, Tw,w_wheel)
Tb = Tbcap * v/(abs(v)+0.001);
end

% wrong, more logic needs to be added to this
% try to find where to incorporate Tw and w_wheel into function

== matlab function P4_Model_2/CarLateralDynamicsBodyFrame/TireSlip ==
  data: vy input size=1; vx input; delta_f input size=1; omega input; alpha_f output; obj parameter; alpha_r output
function [alpha_f, alpha_r] = fcn(vy,  vx, delta_f, omega, obj)


if abs(vx)> obj.vx_threshold1
      alpha_f = delta_f - (vy + omega * obj.lf) / vx;
      alpha_r = - (vy - omega * obj.lr) / vx;
else
      alpha_f = 0;
      alpha_r = 0;
end



end
